simulink model "template"  (Simulink 7.4)
settings: Solver=ode45  StartTime=0.0  StopTime=10.0  RelTol=1e-3
values from neighbouring files (symbols this model uses):
  B = ones(n_states,n_inputs)    [create_ss_model.m]
  C = eye(n_outputs,n_states)    [create_ss_model.m]
  D = diag(diag(M))    [any_matrix_to_elist.m]    (also in create_ss_model.m = zeros(n_outputs,n_inputs))
undefined symbols (not defined in the file or in its folder): Anode
settings Model: Creator=chepeadan  LastModifiedBy=chepeadan

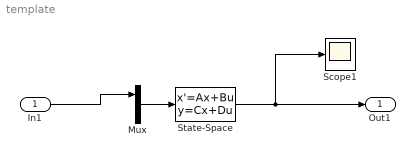
== system template ==
  In1 : Inport  OutDataType=fixdt(1, 16)  OutScaling=2^0
  Mux : Mux  Inputs=2
  Scope1 : Scope
      settings: TimeRange=0.5847953216374258  YMin=-0.1657458563535892  YMax=1.21546961325967
  State-Space : StateSpace  A=Anode  B=B  C=C  D=D  X0=10
  Out1 : Outport  OutDataType=fixdt(1, 16)  OutScaling=2^0
  wires:
  Mux/1 -> State-Space/1
  In1/1 -> Mux/1
  State-Space/1 -> Out1/1, Scope1/1
